simulink model "ServoMotor_Model"  (R2015a)
settings: Solver=ode45  StartTime=0.0  StopTime=10.0  RelTol=1e-3
undefined symbols (not defined in the file): B0, B1, B2, B3, degtorad, m_servo, q_servo, ServoMotor_Gain, sigbuilder_block
settings Model: Creator=Claudio  LastModifiedBy=Claudio

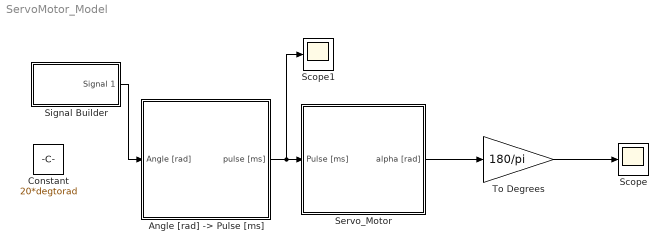
== system ServoMotor_Model ==
  "Angle [rad] -> Pulse [ms]" : Subsystem
  Constant : Constant  Value=20*degtorad
  Scope : Scope
  Scope1 : Scope
  Servo_Motor : Subsystem
  Signal Builder : Subsystem  Tag=STV Subsys  LoadFcn=sigbuilder_block('load');  StartFcn=sigbuilder_block('start');  StopFcn=sigbuilder_block('stop');  ClipboardFcn=sigbuilder_block('clipboard');  mask(Sigbuilder block){}
      mask help: Simulink:masks:SigbuilderBlock_MD
      mask init:
      | if ~strcmp(get_param(bdroot(gcbh),'SimulationStatus'),'stopped') tuvar = sigbuilder_block('maskInit'); end
      settings: CopyFcn=sigbuilder_block('copy');  DeleteFcn=sigbuilder_block('delete');  ModelCloseFcn=sigbuilder_block('modelClose');  PreSaveFcn=sigbuilder_block('preSave');  PauseFcn=sigbuilder_block('pause');  ContinueFcn=sigbuilder_block('continue');  NameChangeFcn=sigbuilder_block('namechange');  OpenFcn=sigbuilder_block('open',[437.6 199.2 550.4 400 ]);  CloseFcn=sigbuilder_block('close');
      mask Display: plot(0, 0, 100, 100,[2, 2, 32, 32, 2], [68, 8, 8, 68, 68],[32, 2], [38, 38], [32, 19, 2],[53, 60, 44], [32, 17, 17, 2],[16, 16, 31, 31]);txt = getActiveGroup(gcbh);text(2, 100, txt,'verticalAlignment', 'top');
  To Degrees : Gain  Gain=180/pi
  wires:
  Servo_Motor/1(alpha [rad]) -> To Degrees/1
  To Degrees/1 -> Scope/1
  "Angle [rad] -> Pulse [ms]"/1(pulse [ms]) -> Scope1/1, Servo_Motor/1(Pulse [ms])
  Signal Builder/1(Signal 1) -> "Angle [rad] -> Pulse [ms]"/1(Angle [rad])

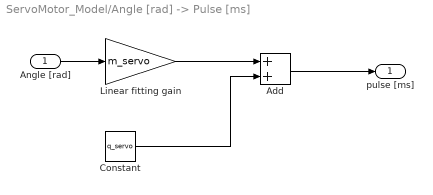
== system ServoMotor_Model/Angle [rad] -> Pulse [ms] ==
  Angle [rad] : Inport
  Add : Sum
  Constant : Constant  Value=q_servo
  Linear fitting gain : Gain  Gain=m_servo
  pulse [ms] : Outport
  wires:
  Angle [rad]/1 -> Linear fitting gain/1
  Constant/1 -> Add/2
  Linear fitting gain/1 -> Add/1
  Add/1 -> pulse [ms]/1

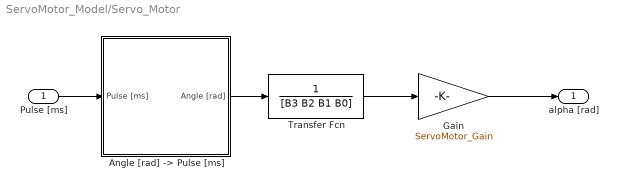
== system ServoMotor_Model/Servo_Motor ==
  Pulse [ms] : Inport
  "Angle [rad] -> Pulse [ms]" : Subsystem
  Gain : Gain  Gain=ServoMotor_Gain
  Transfer Fcn : TransferFcn  Denominator=[B3 B2 B1 B0]
  alpha [rad] : Outport
  wires:
  Gain/1 -> alpha [rad]/1
  Transfer Fcn/1 -> Gain/1
  "Angle [rad] -> Pulse [ms]"/1(Angle [rad]) -> Transfer Fcn/1
  Pulse [ms]/1 -> "Angle [rad] -> Pulse [ms]"/1(Pulse [ms])

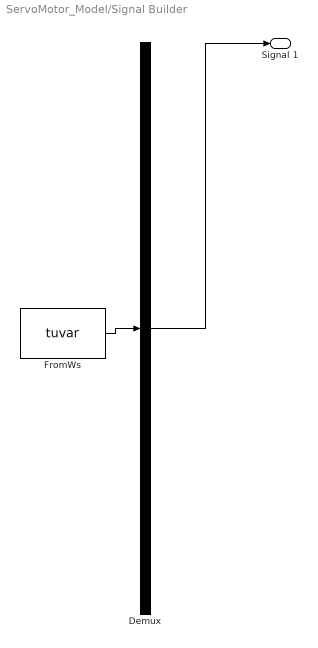
== system ServoMotor_Model/Signal Builder ==
  Demux : Demux  Tag=STV Demux  Outputs=1
  FromWs : FromWorkspace  Tag=STV FromWs  VariableName=tuvar  SampleTime=0
      SigBuilderData=|
      | common.afterFinalStr = 'Extrapolate'
      | common.sampleTime = 0
      | dataSet.timeRange = [0 10]
      | dataSet.name = 'Group 1'
      | sbobj.Groups.Name = 'Group 1'
      | sbobj.Groups.Signals.Name = 'Signal 1'
      | sbobj.Groups.Signals.XData = [0 0.8 0.8 1.6 1.6 2.4 2.4 3.2 3.2 10]
      | sbobj.Groups.Signals.YData = [0 0 0.15 0.15 0 0 0.15 0.15 0 0]
  Signal 1 : Outport  Tag=STV Outport
  wires:
  Demux/1 -> Signal 1/1
  FromWs/1 -> Demux/1

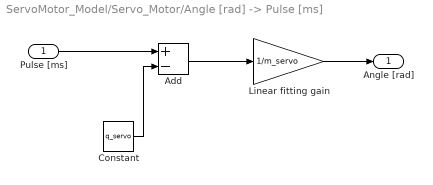
== system ServoMotor_Model/Servo_Motor/Angle [rad] -> Pulse [ms] ==
  Pulse [ms] : Inport
  Add : Sum  Inputs=+-
  Constant : Constant  Value=q_servo
  Linear fitting gain : Gain  Gain=1/m_servo
  Angle [rad] : Outport
  wires:
  Constant/1 -> Add/2
  Add/1 -> Linear fitting gain/1
  Pulse [ms]/1 -> Add/1
  Linear fitting gain/1 -> Angle [rad]/1
